simulink model "stm32f0_motor_control_demo"  (Simulink 7.3)
settings: Solver=ode3  SolverMode=SingleTasking  StartTime=0.0  StopTime=10.0  RelTol=1e-3
PreLoadFcn:
  | waijung.modelPreload; % Required for working with Waijung Blockset. Do not remove.
undefined symbols (not defined in the file): current, Da1, Da2, Db1, Db2, EN1, EN2, LQFP48, STM32F072CB, voltage
libraries: stm32f0_io_lib x4, stm32f0_adc_lib x1, stm32f0_device_config_lib x1
CloseFcn:
  | waijung.modelClose; % Required for working with Waijung Blockset. Do not remove.
settings Model: Creator=Krisada  LastModifiedBy=Krisada
settings OptimizationCC: OptimizeModelRefInitCode=on  LifeSpan=1
settings HardwareCC: ProdEndianess=LittleEndian  ProdHWDeviceType=ARM Compatible->Cortex - M0  TargetEndianess=LittleEndian  TargetHWDeviceType=ARM Compatible->Cortex - M0
settings RTWCC: SystemTargetFile=stm32f0.tlc  GenerateMakefile=off  TemplateMakefile=ert_default_tmf  Description=STM32F0 Target  ProcessScript=stm32f0_make_rtw_hook
settings CodeAppCC: IgnoreCustomStorageClasses=off
settings STFCustomTargetCC: ModelReferenceCompliant=off  CombineOutputUpdateFcns=on  ERTCustomFileBanners=on  SupportContinuousTime=off  SupportNonInlinedSFcns=off  SystemTargetFile=stm32f0.tlc
settings ERTTargetCC: MultiwordLength=2048  ModelReferenceCompliant=off  ParMdlRefBuildCompliant=off  CompOptLevelCompliant=off  ERTFirstTimeCompliant=off  ModelStepFunctionPrototypeControlCompliant=off  CPPClassGenCompliant=off  InlinedParameterPlacement=NonHierarchical  ERTSrcFileBannerTemplate=stm32f0_code_template.cgt  ERTHdrFileBannerTemplate=stm32f0_code_template.cgt  ERTDataSrcFileTemplate=stm32f0_code_template.cgt  ERTDataHdrFileTemplate=stm32f0_code_template.cgt  ERTCustomFileTemplate=stm32f0_file_process.tlc

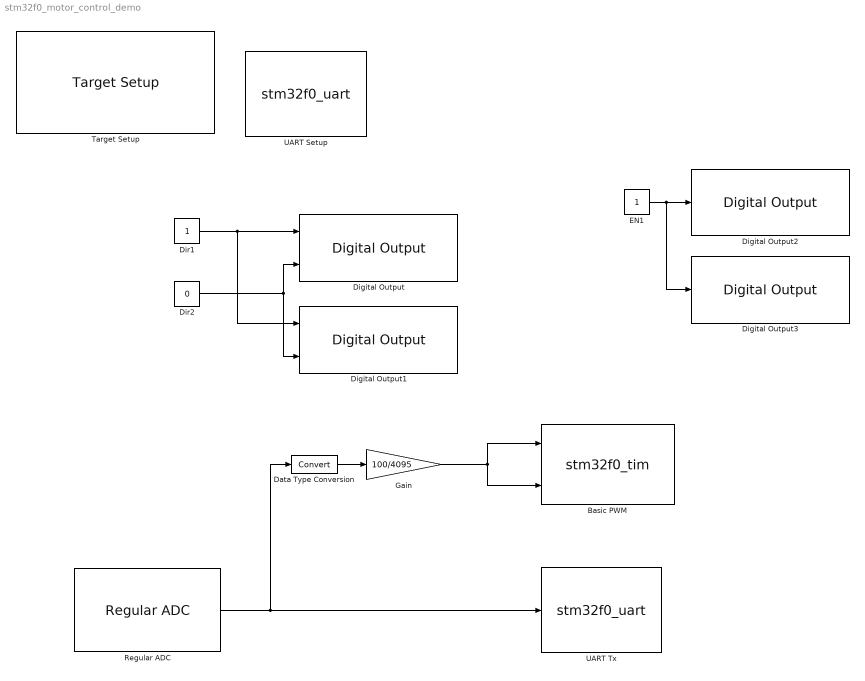
== system stm32f0_motor_control_demo ==
  Basic PWM : S-Function  FunctionName=stm32f0_tim  Parameters=conf,inputporttype,inputportwidth,outputporttype,outputportwidth,optionstring,sampletime,blockid  EnableBusSupport=off  mask(stm32f0_tim){conf=pwm, timer=3, period=0.0001, polarity=Active High, ch1pin=Not available - Do not use, ch2pin=Not available - Do not use, ch3pin=B0, ch4pin=B1, sampletime=inf, enablecustomportlabel=off, cinputportlabel=Motor1,Motor2, coutputportlabel=, portpinstr=0, blockid=BasicPWM, inputporttype=[-1 -1], inputportwidth=[], inputportlabel={'CH3(B0)' 'CH4(B1)'}, outputporttype=[], outputportwidth=[], outputportlabel={}, compat=0, optionstring=["3","1","0.0001","Active High","0","0","1","1","","","B","B","","","0","1","0","0","1","1","0","1","0","0","0","4799","0","TIM_OCPolarity_High"]}
      mask prompts: conf "Configuration"; period "PWM Period (seconds)"; ch1pin "Channel 1"; ch2pin "Channel 2"; ch3pin "Channel 3"; ch4pin "Channel 4"; sampletime "Sample time (sec)"; enablecustomportlabel "Enable custom port labels (Ex. In1, In2, In3)"; cinputportlabel "Custom input port labels (Ex. In1, In2, In3)"; coutputportlabel "Custom output port labels (Ex. Out1, Out2, Out3)"; portpinstr "Port Pin String"; blockid "Block ID"; inputporttype "Input Port Type"; inputportwidth "Input Port Width"; inputportlabel "Input Port Label"; outputporttype "Output Port Type"; outputportwidth "Output Port Width"; outputportlabel "Output port label"; compat "Compatibility (Reserved for future use)"; optionstring "String(s) to be passed to TLC"
      mask init:
      | stm32f0_tim_callback('init');
      mask Help: web(fullfile(waijungdocroot,'stm32f0_tim.htm'), '-browser')
      mask StyleString: popup(pwm),popup(1|2|3|14|15|16|17),edit,popup(Active High|Active Low),popup(Not available - Do not use|A6|C6|B4),popup(Not available - Do not use|A7|C7|B5),popup(Not available - Do not use|B0|C8),popup(Not available - Do not use|B1|C9),edit,checkbox,edit,edit,edit,edit,edit,edit,edit,edit,edit,edit,edit,edit
      mask CallbackString: stm32f0_tim_callback('conf');|stm32f0_tim_callback('timer');|||||||stm32f0_tim_callback('sampletime');|stm32f0_tim_callback('enablecustomportlabel');|stm32f0_tim_callback('conf');|stm32f0_tim_callback('conf');||stm32f0_tim_callback('blockid');||||||||
      mask Display: text(0.95, 0.5, 'Timer: 3\nPolarity: Active High\nPeriod (sec): 0.0001\nTs (sec): 0.1','ver','middle','hor','right'); port_label('input', 1,'CH3(B0)'); port_label('input', 2,'CH4(B1)');
  Data Type Conversion : DataTypeConversion  OutDataType=fixdt(1, 16)  OutScaling=2^0
  Digital Output : stm32f0_io_lib/Digital Output  use_bitband=off  port=B  speed=2  porttype=Open Drain  porttypestr=OD  use_pin0=off  use_pin1=off  use_pin2=on  use_pin3=off  use_pin4=off  use_pin5=off  use_pin6=off  use_pin7=off  use_pin8=off  use_pin9=off  use_pin10=off  use_pin11=off  use_pin12=on  use_pin13=off  use_pin14=off  use_pin15=off  pinstr=GPIO_Pin_2 | GPIO_Pin_12  usedpinarray="[0  0  1  0  0  0  0  0  0  0  0  0  1  0  0  0]"  bitbandingstr=|  sampletime=-1  sampletimestr=0.1  blockid=DigitalOutput  enablecustomportlabel=on  cinputportlabel=Db1,Db2,EN2  coutputportlabel=0
      | #define DigitalOutput_B2 Peripheral_BB(GPIOB->ODR, 2)  /* Output pin */
      | #define DigitalOutput_B12 Peripheral_BB(GPIOB->ODR, 12)  /* Output pin */
  Digital Output1 : stm32f0_io_lib/Digital Output  use_bitband=off  port=A  speed=2  porttype=Open Drain  porttypestr=OD  use_pin0=off  use_pin1=off  use_pin2=off  use_pin3=off  use_pin4=off  use_pin5=off  use_pin6=off  use_pin7=off  use_pin8=on  use_pin9=off  use_pin10=off  use_pin11=on  use_pin12=off  use_pin13=off  use_pin14=off  use_pin15=off  pinstr=GPIO_Pin_8 | GPIO_Pin_11  usedpinarray="[0  0  0  0  0  0  0  0  1  0  0  1  0  0  0  0]"  bitbandingstr=|  sampletime=-1  sampletimestr=0.1  blockid=DigitalOutput1  enablecustomportlabel=on  cinputportlabel=Da1,Da2,EN1  coutputportlabel=0
      | #define DigitalOutput1_A8 Peripheral_BB(GPIOA->ODR, 8)  /* Output pin */
      | #define DigitalOutput1_A11 Peripheral_BB(GPIOA->ODR, 11)  /* Output pin */
  Digital Output2 : stm32f0_io_lib/Digital Output  use_bitband=off  port=B  speed=2  porttype=Push Pull  porttypestr=PP  use_pin0=off  use_pin1=off  use_pin2=off  use_pin3=off  use_pin4=off  use_pin5=off  use_pin6=off  use_pin7=off  use_pin8=off  use_pin9=off  use_pin10=off  use_pin11=off  use_pin12=off  use_pin13=on  use_pin14=off  use_pin15=off  pinstr=GPIO_Pin_13  usedpinarray="[0  0  0  0  0  0  0  0  0  0  0  0  0  1  0  0]"  bitbandingstr="#define DigitalOutput2_B13 Peripheral_BB(GPIOB->ODR, 13)  /* Output pin */"  sampletime=-1  sampletimestr=0.1  blockid=DigitalOutput2  enablecustomportlabel=off  cinputportlabel=Db1,Db2,EN2  coutputportlabel=0
  Digital Output3 : stm32f0_io_lib/Digital Output  use_bitband=off  port=A  speed=2  porttype=Push Pull  porttypestr=PP  use_pin0=off  use_pin1=off  use_pin2=off  use_pin3=off  use_pin4=off  use_pin5=off  use_pin6=off  use_pin7=off  use_pin8=off  use_pin9=off  use_pin10=off  use_pin11=off  use_pin12=on  use_pin13=off  use_pin14=off  use_pin15=off  pinstr=GPIO_Pin_12  usedpinarray="[0  0  0  0  0  0  0  0  0  0  0  0  1  0  0  0]"  bitbandingstr="#define DigitalOutput3_A12 Peripheral_BB(GPIOA->ODR, 12)  /* Output pin */"  sampletime=-1  sampletimestr=0.1  blockid=DigitalOutput3  enablecustomportlabel=off  cinputportlabel=Da1,Da2,EN1  coutputportlabel=0
  Dir1 : Constant  OutDataTypeMode=uint8  OutDataType=fixdt(1, 16)  OutScaling=2^0  OutDataTypeStr=uint8
  Dir2 : Constant  Value=0  OutDataTypeMode=uint8  OutDataType=fixdt(1, 16)  OutScaling=2^0  OutDataTypeStr=uint8
  EN1 : Constant  OutDataTypeMode=uint8  OutDataType=fixdt(1, 16)  OutScaling=2^0  OutDataTypeStr=uint8
  Gain : Gain  Gain=100/4095  ParameterDataTypeMode=single  ParameterDataType=fixdt(1, 16)  ParameterScaling=2^0  ParamDataTypeStr=single  OutDataType=fixdt(1, 16)  OutScaling=2^0
  Regular ADC : stm32f0_adc_lib/Regular ADC  conf=adc  module=1  samplingtime=55.5 Cycles  outputdatatype=Uint16  adc_ch0=on  adc_ch1=off  adc_ch2=off  adc_ch3=off  adc_ch4=off  adc_ch5=off  adc_ch6=off  adc_ch7=off  adc_ch8=off  adc_ch9=off  adc_ch10=off  adc_ch11=off  adc_ch12=off  adc_ch13=off  adc_ch14=off  adc_ch15=off  adc_ch16=off  adc_ch17=off  adc_ch18=off  sampletime=inf  enablecustomportlabel=off  coutputportlabel=voltage,current  portpinstr=0  blockid=RegularADC  inputporttype=[]  inputportwidth=[]  inputportlabel={}  outputporttype=[5]  outputportwidth=[]  outputportlabel={'ADC_IN0'}  compat=0  optionstring="[\"1\",\"ADC_SampleTime_55_5Cycles\",\"dummy\",\"dummy\",\"dummy\",\"1\",\"A\",\"0\",\"0\",\"A\",\"1\",\"0\",\"A\",\"2\",\"0\",\"A\",\"3\",\"0\",\"A\",\"4\",\"0\",\"A\",\"5\",\"0\",\"A\",\"6\",\"0\",\"A\",\"7\",\"0\",\"B\",\"0\",\"0\",\"B\",\"1\",\"0\",\"C\",\"0\",\"0\",\"C\",\"1\",\"0\",\"C\",\"2\",\"0\",\"C\",\"3\",\"0\",\"C\",\"4\",\"0\",\"C\",\"5\",\"0\",\"A\",\"0\",\"0\",\"A\",\"0\",\"0\",\"A\",\"0\",\"1\",\"1\",\"1\",\"1\",\"0\",\"0\",\"0\",\"uint16_t\"]"
  Target Setup : stm32f0_device_config_lib/Target Setup  Priority=100  compiler=GNU ARM  previous_compiler=GNU ARM  mcu=STM32F072CB (LQFP48)  mcustr=STM32F072CB  stdlib=STM32F072  clockconfig=STM32F072B-DISCO Default (HSIOSC-8MHz/HCLK-48MHz)  system_stm32f0xx_c_path=F:\trunk\targets\stm32f0_target\stm32f0\utils\STM32F0xx_AN4055\stm32f0_default\hsi8mhz_pll_hclk48mhz  showmemoryconfiguration=on  stacksize=0x400  heapsize=0x200  enableautocompiledownload=on  fullchiperase=off  programmerinterface=aMG USB Connect  editctrlstr=on  compilercontrolstr=$(patsubst %, -I%, .) -mcpu=cortex-m0 -mthumb -mabi=aapcs -Wall -O3 -mfloat-abi=soft -ffunction-sections -fdata-sections -fno-strict-aliasing -fno-builtin --short-enums  assemblercontrolstr=$(patsubst %, -I%, .) -mcpu=cortex-m0 -mtune=cortex-m0 -mthumb -Wall -O3 -Wa,-amhls=$(<:.s=.lst) -D__STACK_SIZE=$(STACK_SIZE) -D__HEAP_SIZE=$(HEAP_SIZE)  linkercontrolstr="-T$(LD_SCRIPT) -Wl,-Map=$(MAP),--cref,--no-warn-mismatch -mcpu=cortex-m0 -mthumb  -Wall -O3 -mabi=aapcs -lc -specs=nosys.specs"  runafterdownload=on  execprofile=None  profileruart=3  profilerbaud=500000  profilertxpin=Not used  profilerinitstr=0.1,48000000,4800000,500000,0  manualsetsampletime=off  sampletime=0.1  blockid=TargetSetup  systickreloadvalue=4800000  hseval=8000000  lastprofileruart=3  hclk=48000000  flashorigin=0x8000000  flashlength=128k  ramorigin=0x20000000  ramlength=16k  useextram=off
  UART Setup : S-Function  FunctionName=stm32f0_uart  Parameters=conf,inputporttype,inputportwidth,outputporttype,outputportwidth,asciiheader,optionstring,headerstring,terminatorstring,asciidatatypestring,sampletime,blockid  EnableBusSupport=off  mask(stm32f0_uart){conf=Setup, uartmodule=1, baudrate=115200, databits=8, parity=No, stopbit=1, remaptxpin=A9, remaprxpin=A10, flowcontrol=None, remapctspin=Not used, remaprtspin=Not used, advanceoptions=on, rxbuffersize=64, txbuffersize=64, transfer=Non-Blocking, packetmode=Binary, binheader='7E 7E', binterminator='03 03', porttype_double=1, porttype_single=1, porttype_int8=0, porttype_uint8=0, porttype_int16=0, porttype_uint16=1, porttype_int32=0, porttype_uint32=0, asciiformat='%1.2f', rx_asciiterminator=CR (0x0D - "\r"), tx_asciiterminator=CR (0x0D - "\r"), storagename=<empty>, varname=, asciiheader=, sampletime=-1, enablecustomportlabel=off, cinputportlabel=de, coutputportlabel=fff,ff,sdfsd, portpinstr=0, blockid=UARTSetup, inputporttype=[], inputportwidth=[], inputportlabel={}, outputporttype=[], outputportwidth=[], outputportlabel={}, compat=0, optionstring=["1", "1", "A", "9", "1", "A", "10", "0", "*", "*", "0", "*", "*", "1", "1", "", "", "115200", "8", "No", "1", "None", "3", "2", "64", "64", "Binary", "Non-Blocking", ""], headerstring=[], terminatorstring=[], asciidatatypestring=[], lastmodule=1}
      mask prompts: conf "Configuration"; uartmodule "UART Module"; baudrate "Baud rate (bps)"; databits "Data bits"; stopbit "Stop bit"; remaptxpin "Tx pin"; remaprxpin "Rx pin"; flowcontrol "Hardware flow control"; remapctspin "HW Flow control, CTS Pin"; remaprtspin "HW Flow control, RTS Pin"; advanceoptions "Advance options"; rxbuffersize "Rx buffer size (bytes)"; txbuffersize "Tx buffer size (bytes)"; packetmode "Packet mode"; binheader "Binary header (example: '7E 7E')"; binterminator "Binary terminator (example: '03 03')"; porttype_double "Number of data port, type DOUBLE"; porttype_single "Number of data port, type SINGLE"; porttype_int8 "Number of data port, type INT8"; porttype_uint8 "Number of data port, type UINT8"; porttype_int16 "Number of data port, type INT16"; porttype_uint16 "Number of data port, type UINT16"; porttype_int32 "Number of data port, type INT32"; porttype_uint32 "Number of data port, type UINT32"; asciiformat "Ascii format"; rx_asciiterminator "End of packet"; tx_asciiterminator "End of packet"; storagename "Buffer"; varname "Var name"; asciiheader "Ascii header (printf format)"; sampletime "Sample time (sec)"; enablecustomportlabel "Enable custom port labels (Ex. In1, In2, In3)"; cinputportlabel "Custom input port labels (Ex. In1, In2, In3)"; coutputportlabel "Custom output port labels (Ex. Out1, Out2, Out3)"; portpinstr "Port Pin String"; blockid "Block ID"; inputporttype "Input Port Type"; inputportwidth "Input Port Width"; inputportlabel "Input Port Label"; outputporttype "Output Port Type"; outputportwidth "Output Port Width"; outputportlabel "Output port label"; compat "Compatibility (Reserved for future use)"; optionstring "String(s) to be passed to TLC"; lastmodule "Last module selected"
      mask help:
      | Default configuration for aMG USB Connect board:
      |  - UART module: 1
      |  - Tx pin: A9
      |  - Rx pin: A10
      |
      | Advance options
      |  - Rx buffer size (bytes): max packet length can be received via DMA.
      |  - Tx buffer size (bytes): max packet length can be transmit via DMA.
      mask init:
      | stm32f0_uart_callback('init');
      mask Help: web(fullfile(waijungdocroot,'stm32f0_uart_setup.htm'), '-browser')
      mask StyleString: popup(Setup|Tx|Rx),popup(1|2|3|4),edit,popup(8),popup(No|Odd|Even),popup(0.5|1|1.5|2),popup(Not used|A9|B6),popup(Not used|A10|B7),popup(None|RTS|CTS|RTS/CTS),popup(Not used|A11),popup(Not used|A12),checkbox,popup(16|32|64|128|256|512),popup(16|32|64|128|256|512),popup(Blocking|Non-Blocking),popup(Ascii|Binary|String Buffer),edit,edit,edit,edit,edit,edit,edit,edit,edit,edit,edit,popup(CR (0x0D - "\r")|LF (0x0A - "\n")|CRLF (0x0D 0x0A - "\r\n")),popup(CR (0x0D - "\r")|LF (0x0A - "\n")|CRLF (0x0D 0x0A - "\r\n")|None),popup(<empty>),edit,edit,edit,checkbox,edit,edit,edit,edit,edit,edit,edit,edit,edit,edit,edit,edit,edit,edit,edit,edit
      mask CallbackString: stm32f0_uart_callback('conf');|stm32f0_uart_callback('uartmodule');|||||||stm32f0_uart_callback('flowcontrol');|||stm32f0_uart_callback('advanceoptions');|||stm32f0_uart_callback('conf');|stm32f0_uart_callback('conf');|stm32f0_uart_callback('binheader');|stm32f0_uart_callback('binterminator');|||||||||stm32f0_uart_callback('asciiformat');|||stm32f0_uart_callback('storagename');|||stm32f0_uart_callback('sampletime');|stm32f0_uart_callback('enablecustomportlabel');|stm32f0_uart_callback('conf');|stm32f0_uart_callback('conf');||stm32f0_uart_callback('blockid');||||||||||||
      mask Display: text(0.5, 0.5, 'Module: USART1_Setup\nBaud (Bps): 115200\nDMA Buffer: 64/64\nTx/Rx Pin: A9/A10','ver','middle','hor','center');
  UART Tx : S-Function  FunctionName=stm32f0_uart  Parameters=conf,inputporttype,inputportwidth,outputporttype,outputportwidth,asciiheader,optionstring,headerstring,terminatorstring,asciidatatypestring,sampletime,blockid  EnableBusSupport=off  mask(stm32f0_uart){conf=Tx, uartmodule=1, baudrate=115200, databits=8, parity=No, stopbit=1, remaptxpin=A9, remaprxpin=A10, flowcontrol=None, remapctspin=Not used, remaprtspin=Not used, advanceoptions=off, rxbuffersize=64, txbuffersize=64, transfer=Non-Blocking, packetmode=Ascii, binheader='7E 7E', binterminator='03 03', porttype_double=0, porttype_single=0, porttype_int8=0, porttype_uint8=0, porttype_int16=0, porttype_uint16=0, porttype_int32=0, porttype_uint32=2, asciiformat='Value=%u', rx_asciiterminator=CR (0x0D - "\r"), tx_asciiterminator=CRLF (0x0D 0x0A - "\r\n"), storagename=<empty>, varname=, asciiheader=Value=%u\r\n, sampletime=inf, enablecustomportlabel=off, cinputportlabel=de, coutputportlabel=fff,ff,sdfsd, portpinstr=0, blockid=UARTTx, inputporttype=[ -1], inputportwidth=[], inputportlabel={ '%u'}, outputporttype=[], outputportwidth=[], outputportlabel={}, compat=0, optionstring=["1", "1", "A", "9", "1", "A", "10", "0", "*", "*", "0", "*", "*", "1", "1", "", "", "115200", "8", "No", "1", "None", "3", "2", "64", "64", "Ascii", "Non-Blocking", ""], headerstring=[], terminatorstring=["13","10"], asciidatatypestring=["uint32_t"], lastmodule=1}
      mask prompts: conf "Configuration"; uartmodule "UART Module"; baudrate "Baud rate (bps)"; databits "Data bits"; stopbit "Stop bit"; remaptxpin "Tx pin"; remaprxpin "Rx pin"; flowcontrol "Hardware flow control"; remapctspin "HW Flow control, CTS Pin"; remaprtspin "HW Flow control, RTS Pin"; advanceoptions "Advance options"; rxbuffersize "Rx buffer size (bytes)"; txbuffersize "Tx buffer size (bytes)"; packetmode "Packet mode"; binheader "Binary header (example: '7E 7E')"; binterminator "Binary terminator (example: '03 03')"; porttype_double "Number of data port, type DOUBLE"; porttype_single "Number of data port, type SINGLE"; porttype_int8 "Number of data port, type INT8"; porttype_uint8 "Number of data port, type UINT8"; porttype_int16 "Number of data port, type INT16"; porttype_uint16 "Number of data port, type UINT16"; porttype_int32 "Number of data port, type INT32"; porttype_uint32 "Number of data port, type UINT32"; asciiformat "Ascii format"; rx_asciiterminator "End of packet"; tx_asciiterminator "End of packet"; storagename "Buffer"; varname "Var name"; asciiheader "Ascii header (printf format)"; sampletime "Sample time (sec)"; enablecustomportlabel "Enable custom port labels (Ex. In1, In2, In3)"; cinputportlabel "Custom input port labels (Ex. In1, In2, In3)"; coutputportlabel "Custom output port labels (Ex. Out1, Out2, Out3)"; portpinstr "Port Pin String"; blockid "Block ID"; inputporttype "Input Port Type"; inputportwidth "Input Port Width"; inputportlabel "Input Port Label"; outputporttype "Output Port Type"; outputportwidth "Output Port Width"; outputportlabel "Output port label"; compat "Compatibility (Reserved for future use)"; optionstring "String(s) to be passed to TLC"; lastmodule "Last module selected"
      mask help:
      | UART Module
      |  - Select module corresponding to "UART Setup" block.
      | Transfer
      |  - Blocking: after write DMA buffer, the block wait until buffer empty.
      |  - Non-Blocking: the block will not wait for buffer empty.
      | Packet mode:
      |  - Ascii: sending data is ascii, Ascii format + End of packet.
      |  - Binary: sending data is binary format, Header + Data + Terminator
      |  - String Buffer: Volatile Data Storage variable name as sending data.
      | Ascii format:
      |  - %U, %I, %D, %O, %X, %u, %i, %d, %o, %x: Uint32
      |  - %E, %G, %F, %e, %g, %f: Single
      |  - %C, %c: Int8
      |  - %S, %s: (char *), this port is output of Volatile Data Storage Read block, which data type is string.
      mask init:
      | stm32f0_uart_callback('init');
      mask Help: web(fullfile(waijungdocroot,'stm32f0_uart_tx.htm'), '-browser')
      mask StyleString: popup(Setup|Tx|Rx),popup(1|2|3|4),edit,popup(8),popup(No|Odd|Even),popup(0.5|1|1.5|2),popup(Not used|A9|B6),popup(Not used|A10|B7),popup(None|RTS|CTS|RTS/CTS),popup(Not used|A11),popup(Not used|A12),checkbox,popup(16|32|64|128|256|512),popup(16|32|64|128|256|512),popup(Blocking|Non-Blocking),popup(Ascii|Binary|String Buffer),edit,edit,edit,edit,edit,edit,edit,edit,edit,edit,edit,popup(CR (0x0D - "\r")|LF (0x0A - "\n")|CRLF (0x0D 0x0A - "\r\n")),popup(CR (0x0D - "\r")|LF (0x0A - "\n")|CRLF (0x0D 0x0A - "\r\n")|None),popup(<empty>),edit,edit,edit,checkbox,edit,edit,edit,edit,edit,edit,edit,edit,edit,edit,edit,edit,edit,edit,edit,edit
      mask CallbackString: stm32f0_uart_callback('conf');|stm32f0_uart_callback('uartmodule');|||||||stm32f0_uart_callback('flowcontrol');|||stm32f0_uart_callback('advanceoptions');|||stm32f0_uart_callback('conf');|stm32f0_uart_callback('conf');|stm32f0_uart_callback('binheader');|stm32f0_uart_callback('binterminator');|||||||||stm32f0_uart_callback('asciiformat');|||stm32f0_uart_callback('storagename');|||stm32f0_uart_callback('sampletime');|stm32f0_uart_callback('enablecustomportlabel');|stm32f0_uart_callback('conf');|stm32f0_uart_callback('conf');||stm32f0_uart_callback('blockid');||||||||||||
      mask Display: text(0.95, 0.5, 'Module: USART1_Tx\nPacket: Ascii\nTransfer: Non-Blocking\nTs (sec): 0.1','ver','middle','hor','right'); port_label('input', 1,'%u');
  wires:
  Regular ADC/1 -> UART Tx/1, Data Type Conversion/1
  Dir1/1 -> Digital Output/1, Digital Output1/1
  Dir2/1 -> Digital Output/2, Digital Output1/2
  Gain/1 -> Basic PWM/1, Basic PWM/2
  EN1/1 -> Digital Output2/1, Digital Output3/1
  Data Type Conversion/1 -> Gain/1
